simulink model "seat_heating_controller"  (R2022b)
settings: Solver=FixedStepDiscrete  StartTime=0.0  StopTime=inf  RelTol=1e-3
PreLoadFcn:
  | if exist('tl_preloadfcn','file'), tl_preloadfcn(gcs,'22.1.0.27'); end
PostLoadFcn:
  | if exist('tl_postloadfcn','file'), tl_postloadfcn(gcs,'22.1.0.27'); end
InitFcn:
  | if exist('tlds_init','file'), tlds_init(gcs); end
StartFcn:
  | if exist('tlds_start','file'), tlds_start(gcs); end
StopFcn:
  | if exist('tlds_stop','file'), tlds_stop(gcs); end
undefined symbols (not defined in the file or in its folder): TemperatureRanges_TemperatureStage1, TemperatureRanges_TemperatureStage2, TemperatureRanges_TemperatureStage3
libraries: tllib x4
PreSaveFcn:
  | if exist('tl_presavefcn','file'), tl_presavefcn(gcs); end
CloseFcn:
  | if exist('tl_closefcn','file'), tl_closefcn(gcs); end
settings Model: TL_MAIN_DATA={'date',738672.43511479162}  TLVersion=22.1.0.27  DS_PROJECTFILE=seat_heating_controller.dd  Creator=developer  LastModifiedBy=developer
settings SolverCC: AlgebraicLoopSolver=TrustRegion
settings OptimizationCC: BlockReduction=off  ConditionallyExecuteInputs=off  OptimizeBlockIOStorage=off
settings DebuggingCC: UnconnectedInputMsg=warning  UnconnectedOutputMsg=warning  UnconnectedLineMsg=warning  BusObjectLabelMismatch=error  StrictBusMsg=ErrorOnBusTreatedAsVector  NonBusSignalsTreatedAsBus=error  SFMachineParentedDataDiag=warning
settings ModelReferenceCC: EnableRefExpFcnMdlSchedulingChecks=on
settings SFSimCC: CustomCodeUndefinedFunction=UseInterfaceOnly

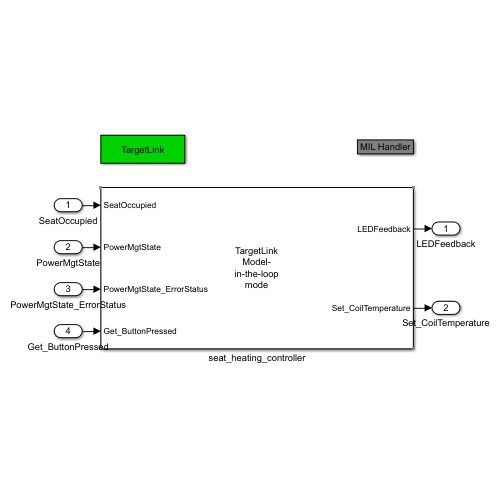
[thumbnail: Simulink's stored preview of the top-level diagram]
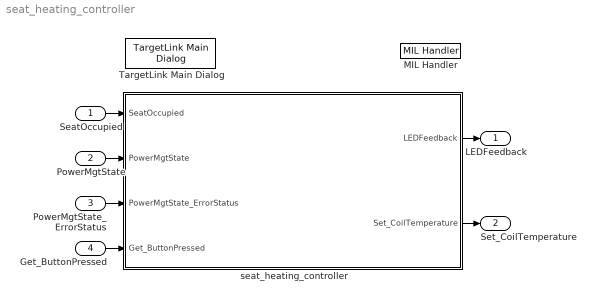
== system seat_heating_controller ==
  SeatOccupied : Inport
  PowerMgtState : Inport  Port=2
  PowerMgtState_ErrorStatus : Inport  Port=3
  Get_ButtonPressed : Inport  Port=4
  MIL Handler : tllib/MIL Handler  data={'date',730486}
      settings: SourceProductName=dSPACE TargetLink common blockset
  TargetLink Main Dialog : tllib/TargetLink Main Dialog  data=[]
      settings: SourceProductName=dSPACE TargetLink common blockset
  seat_heating_controller : Subsystem  Tag=TargetLink Simulation Frame  mask(TL_SimFrame){}
      settings: CopyFcn=if exist('tl_copyfcn','file'), tl_copyfcn(gcbh); end  NameChangeFcn=if exist('tl_framenamechangefcn','file'), tl_framenamechangefcn(gcbh); end
      settings: OpenFcn=|
      | if exist('open_tlsubsystem','file')
      |    open_tlsubsystem(gcbh);
      | else
      |    tlsubsystem = ...
      |       find_system(gcb, ...
      |       'LookUnderMasks','on', ...
      |       'FollowLinks','on', ...
      |       'Tag','MIL Subsystem');
      |    open_system(tlsubsystem);
      | end
      mask Display: disp('TargetLink\nModel-\nin-the-loop\nmode')
  LEDFeedback : Outport
  Set_CoilTemperature : Outport  Port=2
  wires:
  seat_heating_controller/1(LEDFeedback) -> LEDFeedback/1
  PowerMgtState/1 -> seat_heating_controller/2(PowerMgtState)
  seat_heating_controller/2(Set_CoilTemperature) -> Set_CoilTemperature/1
  SeatOccupied/1 -> seat_heating_controller/1(SeatOccupied)
  Get_ButtonPressed/1 -> seat_heating_controller/4(Get_ButtonPressed)
  PowerMgtState_ErrorStatus/1 -> seat_heating_controller/3(PowerMgtState_ErrorStatus)

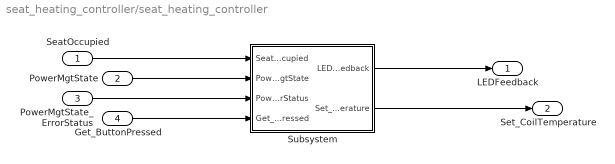
== system seat_heating_controller/seat_heating_controller ==
  SeatOccupied : Inport
  PowerMgtState : Inport  Port=2  OutDataTypeStr=Enum: IDT_PowerState
  PowerMgtState_ErrorStatus : Inport  Port=3
  Get_ButtonPressed : Inport  Port=4
  Subsystem : Subsystem  mask(TL_Enable){}
      settings: OpenFcn=warndlg(get_param(gcb,'MaskHelp'),'Serious Warning');
      mask Help: This subsystem keeps the TargetLink subsystem (subsystem with TargetLink blocks for production code generation), and is needed for the TargetLink simulation frame to work properly. DO NOT DELETE OR MODIFY IT!
  LEDFeedback : Outport  VectorParamsAs1DForOutWhenUnconnected=off
  Set_CoilTemperature : Outport  Port=2  VectorParamsAs1DForOutWhenUnconnected=off
  wires:
  SeatOccupied/1 -> Subsystem/1(SeatOccupied)
  PowerMgtState/1 -> Subsystem/2(PowerMgtState)
  PowerMgtState_ErrorStatus/1 -> Subsystem/3(PowerMgtState_ErrorStatus)
  Get_ButtonPressed/1 -> Subsystem/4(Get_ButtonPressed)
  Subsystem/1(LEDFeedback) -> LEDFeedback/1
  Subsystem/2(Set_CoilTemperature) -> Set_CoilTemperature/1

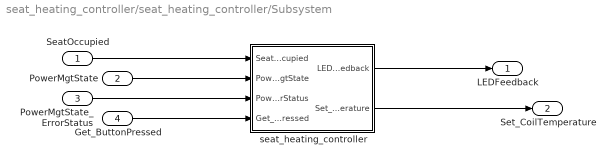
== system seat_heating_controller/seat_heating_controller/Subsystem ==
  SeatOccupied : Inport
  PowerMgtState : Inport  Port=2
  PowerMgtState_ErrorStatus : Inport  Port=3
  Get_ButtonPressed : Inport  Port=4
  seat_heating_controller : Subsystem  Tag=MIL Subsystem  Description=a  LoadFcn=|
      | if exist('TargetLink.SimFrameHandler.TLSubsystem','class')
      |     TargetLink.SimFrameHandler.TLSubsystem.CreateWatchDog(gcbh);
      | end
      settings: CopyFcn=if exist('tl_copyfcn','file'), tl_copyfcn(gcbh); end  NameChangeFcn=if exist('tl_namechangefcn','file'), tl_namechangefcn(gcbh); end  DestroyFcn=if exist('update_tl_main_dlg','file'), update_tl_main_dlg('TL_subs_display'); end
      mask Display: disp('TargetLink Subsystem')
  LEDFeedback : Outport
  Set_CoilTemperature : Outport  Port=2  VectorParamsAs1DForOutWhenUnconnected=off
  wires:
  SeatOccupied/1 -> seat_heating_controller/1(SeatOccupied)
  PowerMgtState/1 -> seat_heating_controller/2(PowerMgtState)
  PowerMgtState_ErrorStatus/1 -> seat_heating_controller/3(PowerMgtState_ErrorStatus)
  Get_ButtonPressed/1 -> seat_heating_controller/4(Get_ButtonPressed)
  seat_heating_controller/1(LEDFeedback) -> LEDFeedback/1
  seat_heating_controller/2(Set_CoilTemperature) -> Set_CoilTemperature/1

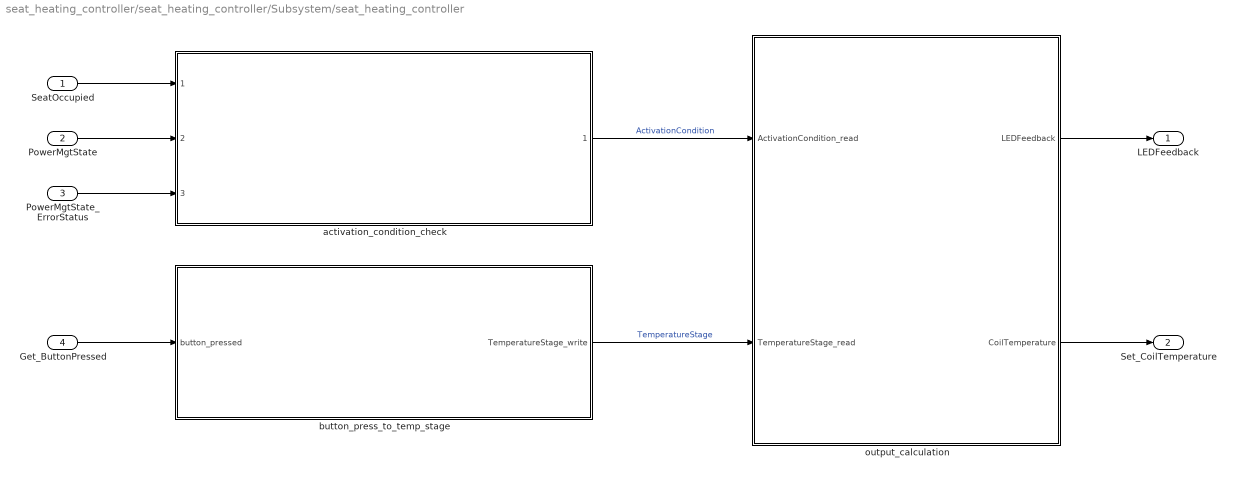
== system seat_heating_controller/seat_heating_controller/Subsystem/seat_heating_controller ==
  SeatOccupied : Inport  PortDimensions=1  mask(TL_Inport){data={'output',{'class','GLOBAL','type','Bool'},'date',738618.42734188656}}
      settings: CopyFcn=if exist('copy_tlblock','file')==2,copy_tlblock(gcbh);end  DeleteFcn=if exist('delete_tlblock','file')==2,delete_tlblock(gcbh);end  NameChangeFcn=if exist('rename_tlblock','file')==2,rename_tlblock(gcbh);end  OpenFcn=if exist('tl_open_blockdlg','file')==2,tl_open_blockdlg(gcbh);else,open_system(gcbh,'force');end
      mask Help: eval(['if exist(''tl_online_help'',''file'') == 2, tl_online_help(''Topic'',''TL_Inport''),else, web([''jar:file:///'',matlabroot,''/help/toolbox/simulink/help.jar!/slref/' lower(get_param(gcbh,'Blocktype')) '.html''], ''-helpbrowser''),end'])
      mask Display:
      | [x,y] = tlDrawBrandOnBlockIcon(gcbh);
      | plot(x,y);
  PowerMgtState : Inport  Port=2  OutDataTypeStr=Enum: IDT_PowerState  PortDimensions=1  mask(TL_Inport){data={'output',{'variable','PowerMgtState'},'date',738618.43935026624}}
      settings: CopyFcn=if exist('copy_tlblock','file')==2,copy_tlblock(gcbh);end  DeleteFcn=if exist('delete_tlblock','file')==2,delete_tlblock(gcbh);end  NameChangeFcn=if exist('rename_tlblock','file')==2,rename_tlblock(gcbh);end  OpenFcn=if exist('tl_open_blockdlg','file')==2,tl_open_blockdlg(gcbh);else,open_system(gcbh,'force');end
      mask Help: eval(['if exist(''tl_online_help'',''file'') == 2, tl_online_help(''Topic'',''TL_Inport''),else, web([''jar:file:///'',matlabroot,''/help/toolbox/simulink/help.jar!/slref/' lower(get_param(gcbh,'Blocktype')) '.html''], ''-helpbrowser''),end'])
      mask Display:
      | [x,y] = tlDrawBrandOnBlockIcon(gcbh);
      | plot(x,y);
  PowerMgtState_ErrorStatus : Inport  Port=3  PortDimensions=1  mask(TL_Inport){data={'output',{'class','GLOBAL','type','UInt8'},'date',738618.43963214115}}
      settings: CopyFcn=if exist('copy_tlblock','file')==2,copy_tlblock(gcbh);end  DeleteFcn=if exist('delete_tlblock','file')==2,delete_tlblock(gcbh);end  NameChangeFcn=if exist('rename_tlblock','file')==2,rename_tlblock(gcbh);end  OpenFcn=if exist('tl_open_blockdlg','file')==2,tl_open_blockdlg(gcbh);else,open_system(gcbh,'force');end
      mask Help: eval(['if exist(''tl_online_help'',''file'') == 2, tl_online_help(''Topic'',''TL_Inport''),else, web([''jar:file:///'',matlabroot,''/help/toolbox/simulink/help.jar!/slref/' lower(get_param(gcbh,'Blocktype')) '.html''], ''-helpbrowser''),end'])
      mask Display:
      | [x,y] = tlDrawBrandOnBlockIcon(gcbh);
      | plot(x,y);
  Get_ButtonPressed : Inport  Port=4  mask(TL_Inport){data={'autosarmode',2,'output',{'class','GLOBAL','type','Bool'},'date',738618.44545436348}}
      settings: CopyFcn=if exist('copy_tlblock') == 2, copy_tlblock(gcbh); end;  DeleteFcn=if exist('delete_tlblock','file')==2,delete_tlblock(gcbh);end  NameChangeFcn=if exist('rename_tlblock','file')==2,rename_tlblock(gcbh);end  OpenFcn=if exist('tl_open_blockdlg','file')==2,tl_open_blockdlg(gcbh);else,open_system(gcbh,'force');end
      mask Help: eval(['if exist(''tl_online_help'',''file'') == 2, tl_online_help(''Topic'',''TL_Inport''),else, web([''jar:file:///'',matlabroot,''/help/toolbox/simulink/help.jar!/slref/' lower(get_param(gcbh,'Blocktype')) '.html''], ''-helpbrowser''),end'])
      mask Display:
      | [x,y] = tlDrawBrandOnBlockIcon(gcbh);
      | plot(x,y);
  activation_condition_check : Subsystem  TreatAsAtomicUnit=on  ReferencedSubsystem=activation_condition_check
  button_press_to_temp_stage : Subsystem  TreatAsAtomicUnit=on
  output_calculation : Subsystem  TreatAsAtomicUnit=on
  LEDFeedback : Outport  PortDimensions=3  mask(TL_Outport){data={'output',{'class','GLOBAL','type','Bool'},'date',738618.44661615742}}
      settings: CopyFcn=if exist('copy_tlblock','file')==2,copy_tlblock(gcbh);end  DeleteFcn=if exist('delete_tlblock','file')==2,delete_tlblock(gcbh);end  NameChangeFcn=if exist('rename_tlblock','file')==2,rename_tlblock(gcbh);end  OpenFcn=if exist('tl_open_blockdlg','file')==2,tl_open_blockdlg(gcbh);else,open_system(gcbh,'force');end
      mask Help: eval(['if exist(''tl_online_help'',''file'') == 2, tl_online_help(''Topic'',''TL_Outport''),else, web([''jar:file:///'',matlabroot,''/help/toolbox/simulink/help.jar!/slref/' lower(get_param(gcbh,'Blocktype')) '.html''], ''-helpbrowser''),end'])
      mask Display:
      | [x,y] = tlDrawBrandOnBlockIcon(gcbh);
      | plot(x,y);
  Set_CoilTemperature : Outport  Port=2  VectorParamsAs1DForOutWhenUnconnected=off  mask(TL_Outport){data={'autosarmode',2,'output',{'class','GLOBAL','type','UInt8'},'date',738618.44780682866}}
      settings: CopyFcn=if exist('copy_tlblock') == 2, copy_tlblock(gcbh); end;  DeleteFcn=if exist('delete_tlblock','file')==2,delete_tlblock(gcbh);end  NameChangeFcn=if exist('rename_tlblock','file')==2,rename_tlblock(gcbh);end  OpenFcn=if exist('tl_open_blockdlg','file')==2,tl_open_blockdlg(gcbh);else,open_system(gcbh,'force');end
      mask Help: eval(['if exist(''tl_online_help'',''file'') == 2, tl_online_help(''Topic'',''TL_Outport''),else, web([''jar:file:///'',matlabroot,''/help/toolbox/simulink/help.jar!/slref/' lower(get_param(gcbh,'Blocktype')) '.html''], ''-helpbrowser''),end'])
      mask Display:
      | [x,y] = tlDrawBrandOnBlockIcon(gcbh);
      | plot(x,y);
  wires:
  SeatOccupied/1 -> activation_condition_check/1
  button_press_to_temp_stage/1(TemperatureStage_write) -> output_calculation/2(TemperatureStage_read)  "TemperatureStage"
  PowerMgtState/1 -> activation_condition_check/2
  output_calculation/1(LEDFeedback) -> LEDFeedback/1
  PowerMgtState_ErrorStatus/1 -> activation_condition_check/3
  activation_condition_check/1 -> output_calculation/1(ActivationCondition_read)  "ActivationCondition"
  Get_ButtonPressed/1 -> button_press_to_temp_stage/1(button_pressed)
  output_calculation/2(CoilTemperature) -> Set_CoilTemperature/1

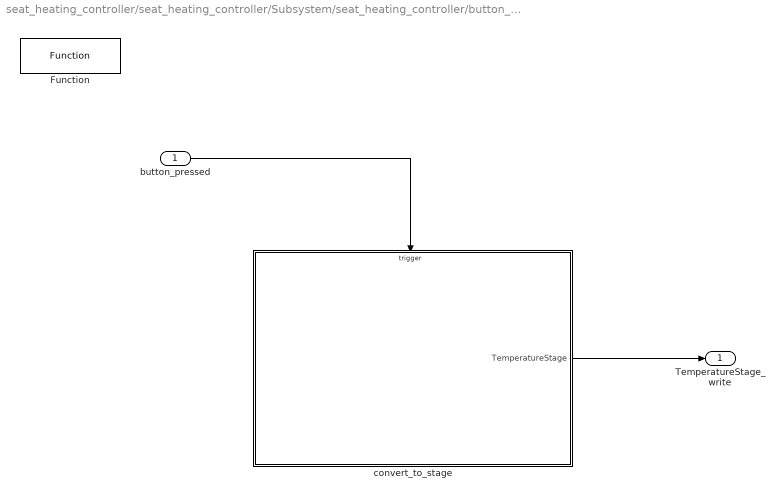
== system seat_heating_controller/seat_heating_controller/Subsystem/seat_heating_controller/button_press_to_temp_stage ==
  button_pressed : Inport
  Function : tllib/Function  data={'date',738618.46715570602}  displayString=FUNCTION
      settings: SourceProductName=dSPACE TargetLink common blockset
  convert_to_stage : Subsystem
  TemperatureStage_write : Outport  OutDataTypeStr=uint8  PortDimensions=1  InitialOutput=0
  wires:
  convert_to_stage/1(TemperatureStage) -> TemperatureStage_write/1
  button_pressed/1 -> convert_to_stage/Trigger

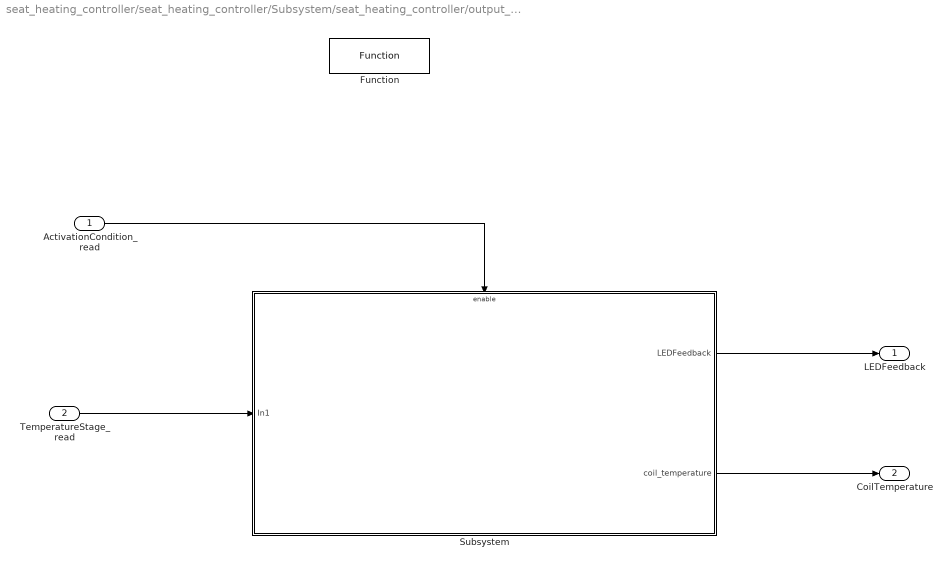
== system seat_heating_controller/seat_heating_controller/Subsystem/seat_heating_controller/output_calculation ==
  ActivationCondition_read : Inport
  TemperatureStage_read : Inport  Port=2
  Function : tllib/Function  data={'date',738618.46736912034}  displayString=FUNCTION
      settings: SourceProductName=dSPACE TargetLink common blockset
  Subsystem : Subsystem
  LEDFeedback : Outport
      settings: EnsureOutportIsVirtual=on
  CoilTemperature : Outport  Port=2  VectorParamsAs1DForOutWhenUnconnected=off
  wires:
  ActivationCondition_read/1 -> Subsystem/Enable
  TemperatureStage_read/1 -> Subsystem/1(In1)
  Subsystem/1(LEDFeedback) -> LEDFeedback/1
  Subsystem/2(coil_temperature) -> CoilTemperature/1

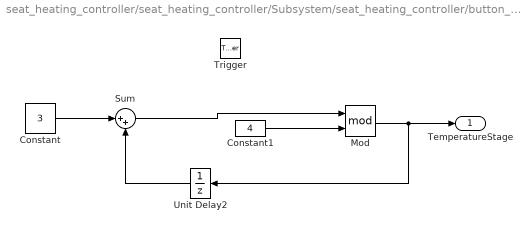
== system seat_heating_controller/seat_heating_controller/Subsystem/seat_heating_controller/button_press_to_temp_stage/convert_to_stage ==
  Trigger : TriggerPort  VariantControl=Variant  PortDimensions=1
  Constant : Constant  Value=3  OutDataTypeStr=Inherit: Inherit via back propagation  mask(TL_Constant){data={'date',739716.74336707173}}
      settings: CopyFcn=if exist('copy_tlblock','file')==2,copy_tlblock(gcbh);end  DeleteFcn=if exist('delete_tlblock','file')==2,delete_tlblock(gcbh);end  NameChangeFcn=if exist('rename_tlblock','file')==2,rename_tlblock(gcbh);end  OpenFcn=if exist('tl_open_blockdlg','file')==2,tl_open_blockdlg(gcbh);else,open_system(gcbh,'force');end
      mask Help: eval(['if exist(''tl_online_help'',''file'') == 2, tl_online_help(''Topic'',''TL_Constant''),else, web([''jar:file:///'',matlabroot,''/help/toolbox/simulink/help.jar!/slref/' lower(get_param(gcbh,'Blocktype')) '.html''], ''-helpbrowser''),end'])
      mask Display:
      | [x,y] = tlDrawBrandOnBlockIcon(gcbh);
      | plot(x,y);
  Constant1 : Constant  Value=4  OutDataTypeStr=Inherit: Inherit via back propagation  mask(TL_Constant){data={'date',739711.94262635417}}
      settings: CopyFcn=if exist('copy_tlblock','file')==2,copy_tlblock(gcbh);end  DeleteFcn=if exist('delete_tlblock','file')==2,delete_tlblock(gcbh);end  NameChangeFcn=if exist('rename_tlblock','file')==2,rename_tlblock(gcbh);end  OpenFcn=if exist('tl_open_blockdlg','file')==2,tl_open_blockdlg(gcbh);else,open_system(gcbh,'force');end
      mask Help: eval(['if exist(''tl_online_help'',''file'') == 2, tl_online_help(''Topic'',''TL_Constant''),else, web([''jar:file:///'',matlabroot,''/help/toolbox/simulink/help.jar!/slref/' lower(get_param(gcbh,'Blocktype')) '.html''], ''-helpbrowser''),end'])
      mask Display:
      | [x,y] = tlDrawBrandOnBlockIcon(gcbh);
      | plot(x,y);
  Mod : Math  Operator=mod  mask(TL_Math){data={'output',{'type','UInt8'},'date',739716.74327490747}}
      settings: CopyFcn=if exist('copy_tlblock','file')==2,copy_tlblock(gcbh);end  DeleteFcn=if exist('delete_tlblock','file')==2,delete_tlblock(gcbh);end  NameChangeFcn=if exist('rename_tlblock','file')==2,rename_tlblock(gcbh);end  OpenFcn=if exist('tl_open_blockdlg','file')==2,tl_open_blockdlg(gcbh);else,open_system(gcbh,'force');end
      mask Help: eval(['if exist(''tl_online_help'',''file'') == 2, tl_online_help(''Topic'',''TL_Math''),else, web([''jar:file:///'',matlabroot,''/help/toolbox/simulink/help.jar!/slref/' lower(get_param(gcbh,'Blocktype')) '.html''], ''-helpbrowser''),end'])
      mask Display:
      | [x,y] = tlDrawBrandOnBlockIcon(gcbh);
      | plot(x,y);
  Sum : Sum  Inputs=|++  mask(TL_Sum){data={'output',{'type','UInt8'},'date',738618.47161409725}}
      settings: CopyFcn=if exist('copy_tlblock','file')==2,copy_tlblock(gcbh);end  DeleteFcn=if exist('delete_tlblock','file')==2,delete_tlblock(gcbh);end  NameChangeFcn=if exist('rename_tlblock','file')==2,rename_tlblock(gcbh);end  OpenFcn=if exist('tl_open_blockdlg','file')==2,tl_open_blockdlg(gcbh);else,open_system(gcbh,'force');end
      mask Help: eval(['if exist(''tl_online_help'',''file'') == 2, tl_online_help(''Topic'',''TL_Sum''),else, web([''jar:file:///'',matlabroot,''/help/toolbox/simulink/help.jar!/slref/' lower(get_param(gcbh,'Blocktype')) '.html''], ''-helpbrowser''),end'])
      mask Display:
      | [x,y] = tlDrawBrandOnBlockIcon(gcbh);
      | plot(x,y);
  Unit Delay2 : UnitDelay  SampleTime=-1  HasFrameUpgradeWarning=on  mask(TL_UnitDelay){data={'output',{'type','UInt8'},'state',{'type','UInt8'},'date',738618.47173122689}}
      settings: AttributesFormatString=Init = %<InitialCondition>  CopyFcn=if exist('copy_tlblock','file')==2,copy_tlblock(gcbh);end  DeleteFcn=if exist('delete_tlblock','file')==2,delete_tlblock(gcbh);end  NameChangeFcn=if exist('rename_tlblock','file')==2,rename_tlblock(gcbh);end  OpenFcn=if exist('tl_open_blockdlg','file')==2,tl_open_blockdlg(gcbh);else,open_system(gcbh,'force');end
      mask Help: eval(['if exist(''tl_online_help'',''file'') == 2, tl_online_help(''Topic'',''TL_UnitDelay''),else, web([''jar:file:///'',matlabroot,''/help/toolbox/simulink/help.jar!/slref/' lower(get_param(gcbh,'Blocktype')) '.html''], ''-helpbrowser''),end'])
      mask Display:
      | [x,y] = tlDrawBrandOnBlockIcon(gcbh);
      | plot(x,y);
  TemperatureStage : Outport  InitialOutput=0
  wires:
  Mod/1 -> TemperatureStage/1, Unit Delay2/1
  Unit Delay2/1 -> Sum/2
  Constant1/1 -> Mod/2
  Sum/1 -> Mod/1
  Constant/1 -> Sum/1

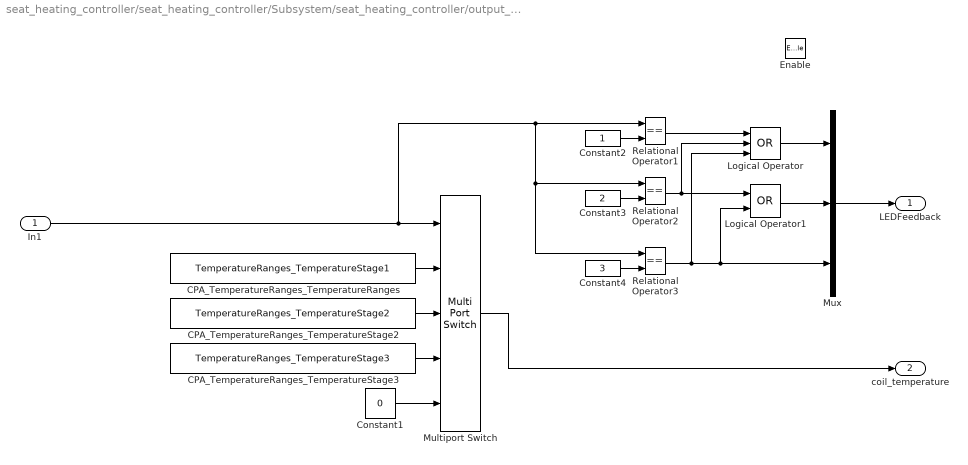
== system seat_heating_controller/seat_heating_controller/Subsystem/seat_heating_controller/output_calculation/Subsystem ==
  In1 : Inport
  Enable : EnablePort
  CPA_TemperatureRanges_TemperatureRanges : Constant  Value=TemperatureRanges_TemperatureStage1  mask(TL_Constant){data={'output',{'class','CAL','type','UInt8'},'date',738618.45283211803}}
      settings: CopyFcn=if exist('copy_tlblock','file')==2,copy_tlblock(gcbh);end  DeleteFcn=if exist('delete_tlblock','file')==2,delete_tlblock(gcbh);end  NameChangeFcn=if exist('rename_tlblock','file')==2,rename_tlblock(gcbh);end  OpenFcn=if exist('tl_open_blockdlg','file')==2,tl_open_blockdlg(gcbh);else,open_system(gcbh,'force');end
      mask Help: eval(['if exist(''tl_online_help'',''file'') == 2, tl_online_help(''Topic'',''TL_Constant''),else, web([''jar:file:///'',matlabroot,''/help/toolbox/simulink/help.jar!/slref/' lower(get_param(gcbh,'Blocktype')) '.html''], ''-helpbrowser''),end'])
      mask Display:
      | [x,y] = tlDrawBrandOnBlockIcon(gcbh);
      | plot(x,y);
  CPA_TemperatureRanges_TemperatureStage2 : Constant  Value=TemperatureRanges_TemperatureStage2  mask(TL_Constant){data={'output',{'class','CAL','type','UInt8'},'date',738618.45289771992}}
      settings: CopyFcn=if exist('copy_tlblock','file')==2,copy_tlblock(gcbh);end  DeleteFcn=if exist('delete_tlblock','file')==2,delete_tlblock(gcbh);end  NameChangeFcn=if exist('rename_tlblock','file')==2,rename_tlblock(gcbh);end  OpenFcn=if exist('tl_open_blockdlg','file')==2,tl_open_blockdlg(gcbh);else,open_system(gcbh,'force');end
      mask Help: eval(['if exist(''tl_online_help'',''file'') == 2, tl_online_help(''Topic'',''TL_Constant''),else, web([''jar:file:///'',matlabroot,''/help/toolbox/simulink/help.jar!/slref/' lower(get_param(gcbh,'Blocktype')) '.html''], ''-helpbrowser''),end'])
      mask Display:
      | [x,y] = tlDrawBrandOnBlockIcon(gcbh);
      | plot(x,y);
  CPA_TemperatureRanges_TemperatureStage3 : Constant  Value=TemperatureRanges_TemperatureStage3  mask(TL_Constant){data={'output',{'class','CAL','type','UInt8'},'date',738618.4529516435}}
      settings: CopyFcn=if exist('copy_tlblock','file')==2,copy_tlblock(gcbh);end  DeleteFcn=if exist('delete_tlblock','file')==2,delete_tlblock(gcbh);end  NameChangeFcn=if exist('rename_tlblock','file')==2,rename_tlblock(gcbh);end  OpenFcn=if exist('tl_open_blockdlg','file')==2,tl_open_blockdlg(gcbh);else,open_system(gcbh,'force');end
      mask Help: eval(['if exist(''tl_online_help'',''file'') == 2, tl_online_help(''Topic'',''TL_Constant''),else, web([''jar:file:///'',matlabroot,''/help/toolbox/simulink/help.jar!/slref/' lower(get_param(gcbh,'Blocktype')) '.html''], ''-helpbrowser''),end'])
      mask Display:
      | [x,y] = tlDrawBrandOnBlockIcon(gcbh);
      | plot(x,y);
  Constant1 : Constant  Value=0  mask(TL_Constant){data={'date',738618.44073870371}}
      settings: CopyFcn=if exist('copy_tlblock','file')==2,copy_tlblock(gcbh);end  DeleteFcn=if exist('delete_tlblock','file')==2,delete_tlblock(gcbh);end  NameChangeFcn=if exist('rename_tlblock','file')==2,rename_tlblock(gcbh);end  OpenFcn=if exist('tl_open_blockdlg','file')==2,tl_open_blockdlg(gcbh);else,open_system(gcbh,'force');end
      mask Help: eval(['if exist(''tl_online_help'',''file'') == 2, tl_online_help(''Topic'',''TL_Constant''),else, web([''jar:file:///'',matlabroot,''/help/toolbox/simulink/help.jar!/slref/' lower(get_param(gcbh,'Blocktype')) '.html''], ''-helpbrowser''),end'])
      mask Display:
      | [x,y] = tlDrawBrandOnBlockIcon(gcbh);
      | plot(x,y);
  Constant2 : Constant  OutDataTypeStr=Inherit: Inherit via back propagation  mask(TL_Constant){data={'date',738618.44073914352}}
      settings: CopyFcn=if exist('copy_tlblock','file')==2,copy_tlblock(gcbh);end  DeleteFcn=if exist('delete_tlblock','file')==2,delete_tlblock(gcbh);end  NameChangeFcn=if exist('rename_tlblock','file')==2,rename_tlblock(gcbh);end  OpenFcn=if exist('tl_open_blockdlg','file')==2,tl_open_blockdlg(gcbh);else,open_system(gcbh,'force');end
      mask Help: eval(['if exist(''tl_online_help'',''file'') == 2, tl_online_help(''Topic'',''TL_Constant''),else, web([''jar:file:///'',matlabroot,''/help/toolbox/simulink/help.jar!/slref/' lower(get_param(gcbh,'Blocktype')) '.html''], ''-helpbrowser''),end'])
      mask Display:
      | [x,y] = tlDrawBrandOnBlockIcon(gcbh);
      | plot(x,y);
  Constant3 : Constant  Value=2  OutDataTypeStr=Inherit: Inherit via back propagation  mask(TL_Constant){data={'date',738618.44073960651}}
      settings: CopyFcn=if exist('copy_tlblock','file')==2,copy_tlblock(gcbh);end  DeleteFcn=if exist('delete_tlblock','file')==2,delete_tlblock(gcbh);end  NameChangeFcn=if exist('rename_tlblock','file')==2,rename_tlblock(gcbh);end  OpenFcn=if exist('tl_open_blockdlg','file')==2,tl_open_blockdlg(gcbh);else,open_system(gcbh,'force');end
      mask Help: eval(['if exist(''tl_online_help'',''file'') == 2, tl_online_help(''Topic'',''TL_Constant''),else, web([''jar:file:///'',matlabroot,''/help/toolbox/simulink/help.jar!/slref/' lower(get_param(gcbh,'Blocktype')) '.html''], ''-helpbrowser''),end'])
      mask Display:
      | [x,y] = tlDrawBrandOnBlockIcon(gcbh);
      | plot(x,y);
  Constant4 : Constant  Value=3  OutDataTypeStr=Inherit: Inherit via back propagation  mask(TL_Constant){data={'date',738618.44074009254}}
      settings: CopyFcn=if exist('copy_tlblock','file')==2,copy_tlblock(gcbh);end  DeleteFcn=if exist('delete_tlblock','file')==2,delete_tlblock(gcbh);end  NameChangeFcn=if exist('rename_tlblock','file')==2,rename_tlblock(gcbh);end  OpenFcn=if exist('tl_open_blockdlg','file')==2,tl_open_blockdlg(gcbh);else,open_system(gcbh,'force');end
      mask Help: eval(['if exist(''tl_online_help'',''file'') == 2, tl_online_help(''Topic'',''TL_Constant''),else, web([''jar:file:///'',matlabroot,''/help/toolbox/simulink/help.jar!/slref/' lower(get_param(gcbh,'Blocktype')) '.html''], ''-helpbrowser''),end'])
      mask Display:
      | [x,y] = tlDrawBrandOnBlockIcon(gcbh);
      | plot(x,y);
  Logical Operator : Logic  Operator=OR  Inputs=3  AllPortsSameDT=off  OutDataTypeStr=boolean  mask(TL_LogicalOperator){data={'date',738618.44074061338}}
      settings: CopyFcn=if exist('copy_tlblock','file')==2,copy_tlblock(gcbh);end  DeleteFcn=if exist('delete_tlblock','file')==2,delete_tlblock(gcbh);end  NameChangeFcn=if exist('rename_tlblock','file')==2,rename_tlblock(gcbh);end  OpenFcn=if exist('tl_open_blockdlg','file')==2,tl_open_blockdlg(gcbh);else,open_system(gcbh,'force');end
      mask Help: eval(['if exist(''tl_online_help'',''file'') == 2, tl_online_help(''Topic'',''TL_LogicalOperator''),else, web([''jar:file:///'',matlabroot,''/help/toolbox/simulink/help.jar!/slref/' lower(get_param(gcbh,'Blocktype')) '.html''], ''-helpbrowser''),end'])
      mask Display:
      | [x,y] = tlDrawBrandOnBlockIcon(gcbh);
      | plot(x,y);
  Logical Operator1 : Logic  Operator=OR  AllPortsSameDT=off  OutDataTypeStr=boolean  mask(TL_LogicalOperator){data={'date',738618.44074107637}}
      settings: CopyFcn=if exist('copy_tlblock','file')==2,copy_tlblock(gcbh);end  DeleteFcn=if exist('delete_tlblock','file')==2,delete_tlblock(gcbh);end  NameChangeFcn=if exist('rename_tlblock','file')==2,rename_tlblock(gcbh);end  OpenFcn=if exist('tl_open_blockdlg','file')==2,tl_open_blockdlg(gcbh);else,open_system(gcbh,'force');end
      mask Help: eval(['if exist(''tl_online_help'',''file'') == 2, tl_online_help(''Topic'',''TL_LogicalOperator''),else, web([''jar:file:///'',matlabroot,''/help/toolbox/simulink/help.jar!/slref/' lower(get_param(gcbh,'Blocktype')) '.html''], ''-helpbrowser''),end'])
      mask Display:
      | [x,y] = tlDrawBrandOnBlockIcon(gcbh);
      | plot(x,y);
  Multiport Switch : MultiPortSwitch  DataPortIndices={0,1,2,3}  DataPortForDefault=Additional data port  DiagnosticForDefault=None  SaturateOnIntegerOverflow=off  InputSameDT=off  mask(TL_MultiPortSwitch){data={'output',{'type','UInt8'},'date',738618.45326392364}}
      settings: CopyFcn=if exist('copy_tlblock','file')==2,copy_tlblock(gcbh);end  DeleteFcn=if exist('delete_tlblock','file')==2,delete_tlblock(gcbh);end  NameChangeFcn=if exist('rename_tlblock','file')==2,rename_tlblock(gcbh);end  OpenFcn=if exist('tl_open_blockdlg','file')==2,tl_open_blockdlg(gcbh);else,open_system(gcbh,'force');end
      mask Help: eval(['if exist(''tl_online_help'',''file'') == 2, tl_online_help(''Topic'',''TL_MultiPortSwitch''),else, web([''jar:file:///'',matlabroot,''/help/toolbox/simulink/help.jar!/slref/' lower(get_param(gcbh,'Blocktype')) '.html''], ''-helpbrowser''),end'])
      mask Display:
      | [x,y] = tlDrawBrandOnBlockIcon(gcbh);
      | plot(x,y);
  Mux : Mux  Inputs=3
  Relational Operator1 : RelationalOperator  Operator===  OutDataTypeStr=boolean  RndMeth=Simplest  InputSameDT=off  mask(TL_RelationalOperator){data={'date',738618.44074226858}}
      settings: CopyFcn=if exist('copy_tlblock','file')==2,copy_tlblock(gcbh);end  DeleteFcn=if exist('delete_tlblock','file')==2,delete_tlblock(gcbh);end  NameChangeFcn=if exist('rename_tlblock','file')==2,rename_tlblock(gcbh);end  OpenFcn=if exist('tl_open_blockdlg','file')==2,tl_open_blockdlg(gcbh);else,open_system(gcbh,'force');end
      mask Help: eval(['if exist(''tl_online_help'',''file'') == 2, tl_online_help(''Topic'',''TL_RelationalOperator''),else, web([''jar:file:///'',matlabroot,''/help/toolbox/simulink/help.jar!/slref/' lower(get_param(gcbh,'Blocktype')) '.html''], ''-helpbrowser''),end'])
      mask Display:
      | [x,y] = tlDrawBrandOnBlockIcon(gcbh);
      | plot(x,y);
  Relational Operator2 : RelationalOperator  Operator===  OutDataTypeStr=boolean  RndMeth=Simplest  InputSameDT=off  mask(TL_RelationalOperator){data={'date',738618.44074277778}}
      settings: CopyFcn=if exist('copy_tlblock','file')==2,copy_tlblock(gcbh);end  DeleteFcn=if exist('delete_tlblock','file')==2,delete_tlblock(gcbh);end  NameChangeFcn=if exist('rename_tlblock','file')==2,rename_tlblock(gcbh);end  OpenFcn=if exist('tl_open_blockdlg','file')==2,tl_open_blockdlg(gcbh);else,open_system(gcbh,'force');end
      mask Help: eval(['if exist(''tl_online_help'',''file'') == 2, tl_online_help(''Topic'',''TL_RelationalOperator''),else, web([''jar:file:///'',matlabroot,''/help/toolbox/simulink/help.jar!/slref/' lower(get_param(gcbh,'Blocktype')) '.html''], ''-helpbrowser''),end'])
      mask Display:
      | [x,y] = tlDrawBrandOnBlockIcon(gcbh);
      | plot(x,y);
  Relational Operator3 : RelationalOperator  Operator===  OutDataTypeStr=boolean  RndMeth=Simplest  InputSameDT=off  mask(TL_RelationalOperator){data={'date',738618.44074325229}}
      settings: CopyFcn=if exist('copy_tlblock','file')==2,copy_tlblock(gcbh);end  DeleteFcn=if exist('delete_tlblock','file')==2,delete_tlblock(gcbh);end  NameChangeFcn=if exist('rename_tlblock','file')==2,rename_tlblock(gcbh);end  OpenFcn=if exist('tl_open_blockdlg','file')==2,tl_open_blockdlg(gcbh);else,open_system(gcbh,'force');end
      mask Help: eval(['if exist(''tl_online_help'',''file'') == 2, tl_online_help(''Topic'',''TL_RelationalOperator''),else, web([''jar:file:///'',matlabroot,''/help/toolbox/simulink/help.jar!/slref/' lower(get_param(gcbh,'Blocktype')) '.html''], ''-helpbrowser''),end'])
      mask Display:
      | [x,y] = tlDrawBrandOnBlockIcon(gcbh);
      | plot(x,y);
  LEDFeedback : Outport
  coil_temperature : Outport  Port=2
  wires:
  In1/1 -> Relational Operator3/1, Relational Operator2/1, Relational Operator1/1, Multiport Switch/1
  Constant2/1 -> Relational Operator1/2
  Constant4/1 -> Relational Operator3/2
  Mux/1 -> LEDFeedback/1
  CPA_TemperatureRanges_TemperatureStage2/1 -> Multiport Switch/3
  Relational Operator2/1 -> Logical Operator1/1, Logical Operator/2
  Relational Operator1/1 -> Logical Operator/1
  Constant3/1 -> Relational Operator2/2
  Relational Operator3/1 -> Logical Operator/3, Logical Operator1/2, Mux/3
  Multiport Switch/1 -> coil_temperature/1
  Constant1/1 -> Multiport Switch/5
  CPA_TemperatureRanges_TemperatureStage3/1 -> Multiport Switch/4
  CPA_TemperatureRanges_TemperatureRanges/1 -> Multiport Switch/2
  Logical Operator/1 -> Mux/1
  Logical Operator1/1 -> Mux/2
